simulink model "spring_damping_system"  (R2017a)
settings: Solver=VariableStepAuto  StartTime=0.0  StopTime=80  RelTol=1e-3
settings Model: Creator=Priyesh  LastModifiedBy=Priyesh

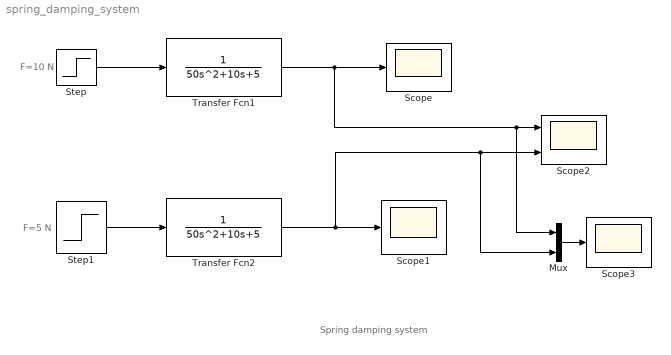
== system spring_damping_system ==
  note: Spring damping system
  note: F=5 N
  note: F=10 N
  Mux : Mux  Inputs=2
  Scope : Scope
  Scope1 : Scope
  Scope2 : Scope  NumInputPorts=2
  Scope3 : Scope
  Step : Step  After=10  SampleTime=0
  Step1 : Step  After=5  SampleTime=0
  Transfer Fcn1 : TransferFcn  Denominator=[50 10 5]
  Transfer Fcn2 : TransferFcn  Denominator=[50 10 5]
  wires:
  Step/1 -> Transfer Fcn1/1
  Step1/1 -> Transfer Fcn2/1
  Transfer Fcn1/1 -> Scope/1, Mux/1, Scope2/1
  Transfer Fcn2/1 -> Scope1/1, Mux/2, Scope2/2
  Mux/1 -> Scope3/1
